simulink model "auv2D_model"  (R2023b)
settings: Solver=FixedStepAuto  StartTime=0.0  StopTime=5  FixedStep=1e-6  RelTol=1e-3
values from neighbouring files (symbols this model uses):
  a1 = Xu/(m-Xud)    (= -0.280372492837)    [auv2D_parameters.m]
  a2 = Yv/(m-Yvd)    (= -0.993417702334)    [auv2D_parameters.m]
  a3 = Nr/(Iz-Nrd)    (= -0.172919127086)    [auv2D_parameters.m]
  b1 = (m-Yvd)/(m-Xud)    (= 2.1006049029)    [auv2D_parameters.m]
  b2 = (Xud-m)/(m-Yvd)    (= -0.4760533495)    [auv2D_parameters.m]
  b3 = (Yvd-Xud)/(Iz-Nrd)    (= -0.887548138639)    [auv2D_parameters.m]
libraries: simulink x1
settings Model: Creator=abinashagasti  LastModifiedBy=abinashagasti

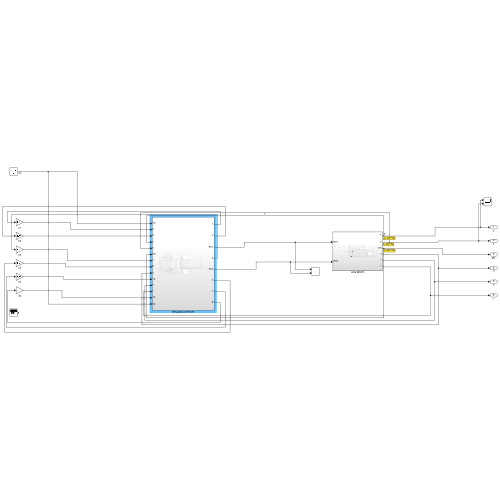
[thumbnail: Simulink's stored preview of the top-level diagram]
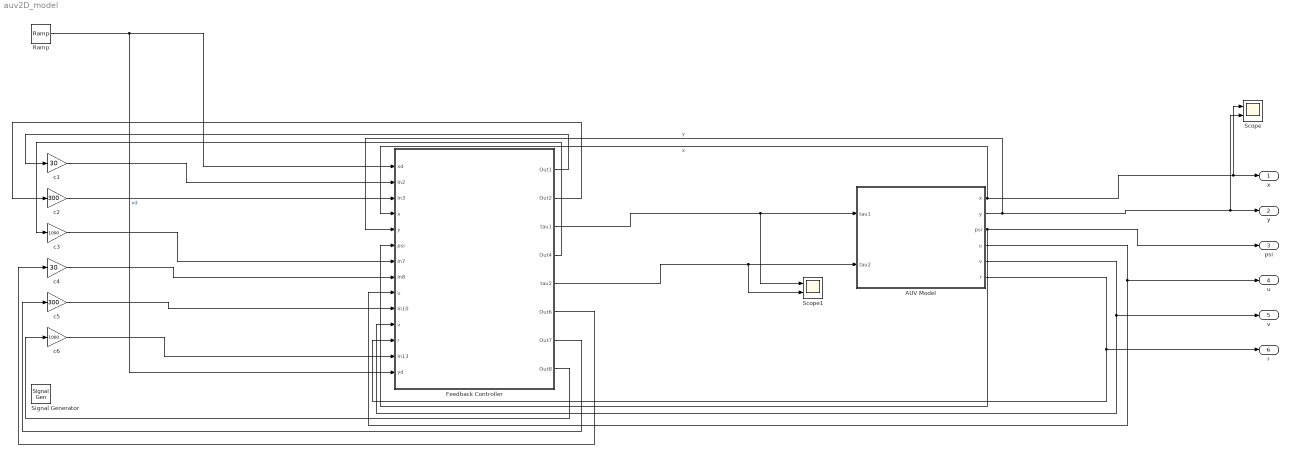
== system auv2D_model ==
  AUV Model : Subsystem
  Feedback Controller : Subsystem
  Ramp : simulink/Sources/Ramp  slope=0.1  start=0  InitialOutput=0
  Scope : Scope  NumInputPorts=2
  Scope1 : Scope  NumInputPorts=2
  Signal Generator : SignalGenerator  Frequency=0.1  Units=rad/sec
  c1 : Gain  Gain=30
  c2 : Gain  Gain=300
  c3 : Gain  Gain=1000
  c4 : Gain  Gain=30
  c5 : Gain  Gain=300
  c6 : Gain  Gain=1000
  x : Outport
  y : Outport  Port=2
  psi : Outport  Port=3
  u : Outport  Port=4
  v : Outport  Port=5
  r : Outport  Port=6
  wires:
  AUV Model/1(x) -> Feedback Controller/4(x), Scope/1, x/1  "x"
  AUV Model/2(y) -> Feedback Controller/5(y), Scope/2, y/1  "y"
  AUV Model/3(psi) -> Feedback Controller/6(psi), psi/1
  AUV Model/4(u) -> Feedback Controller/9(u), u/1
  AUV Model/5(v) -> v/1, Feedback Controller/11(v)
  AUV Model/6(r) -> r/1, Feedback Controller/12(r)
  Ramp/1 -> Feedback Controller/14(yd), Feedback Controller/1(xd)  "xd"
  c1/1 -> Feedback Controller/2(In2)
  c2/1 -> Feedback Controller/3(In3)
  c3/1 -> Feedback Controller/7(In7)
  c4/1 -> Feedback Controller/8(In8)
  c5/1 -> Feedback Controller/10(In10)
  c6/1 -> Feedback Controller/13(In13)
  Feedback Controller/1(Out1) -> c1/1
  Feedback Controller/2(Out2) -> c2/1
  Feedback Controller/3(tau1) -> Scope1/1, AUV Model/1(tau1)
  Feedback Controller/4(Out4) -> c3/1
  Feedback Controller/5(tau2) -> Scope1/2, AUV Model/2(tau2)
  Feedback Controller/6(Out6) -> c4/1
  Feedback Controller/7(Out7) -> c5/1
  Feedback Controller/8(Out8) -> c6/1

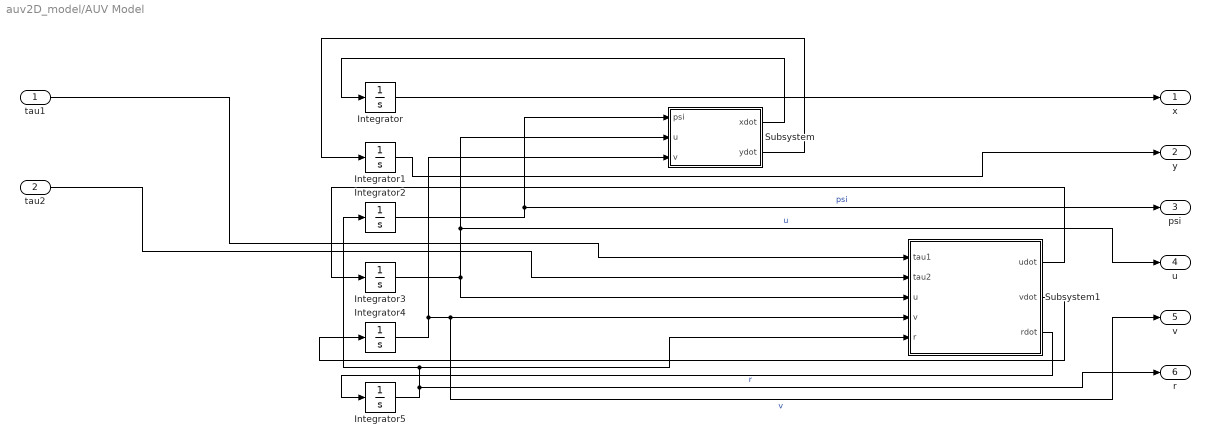
== system auv2D_model/AUV Model ==
  tau1 : Inport
  tau2 : Inport  Port=2
  Integrator{,1,4..5} (4 alike) : Integrator
  Integrator2 : Integrator  InitialCondition=pi/4
  Integrator3 : Integrator  InitialCondition=1
  Subsystem : Subsystem
  Subsystem1 : Subsystem
  x : Outport
  y : Outport  Port=2
  psi : Outport  Port=3
  u : Outport  Port=4
  v : Outport  Port=5
  r : Outport  Port=6
  wires:
  Subsystem1/2(vdot) -> Integrator4/1
  tau2/1 -> Subsystem1/2(tau2)
  Subsystem/2(ydot) -> Integrator1/1
  tau1/1 -> Subsystem1/1(tau1)
  Subsystem1/3(rdot) -> Integrator5/1
  Subsystem1/1(udot) -> Integrator3/1
  Integrator2/1 -> psi/1, Subsystem/1(psi)  "psi"
  Integrator4/1 -> Subsystem/3(v), v/1, Subsystem1/4(v)  "v"
  Integrator1/1 -> y/1
  Subsystem/1(xdot) -> Integrator/1
  Integrator5/1 -> r/1, Subsystem1/5(r), Integrator2/1  "r"
  Integrator/1 -> x/1
  Integrator3/1 -> u/1, Subsystem/2(u), Subsystem1/3(u)  "u"

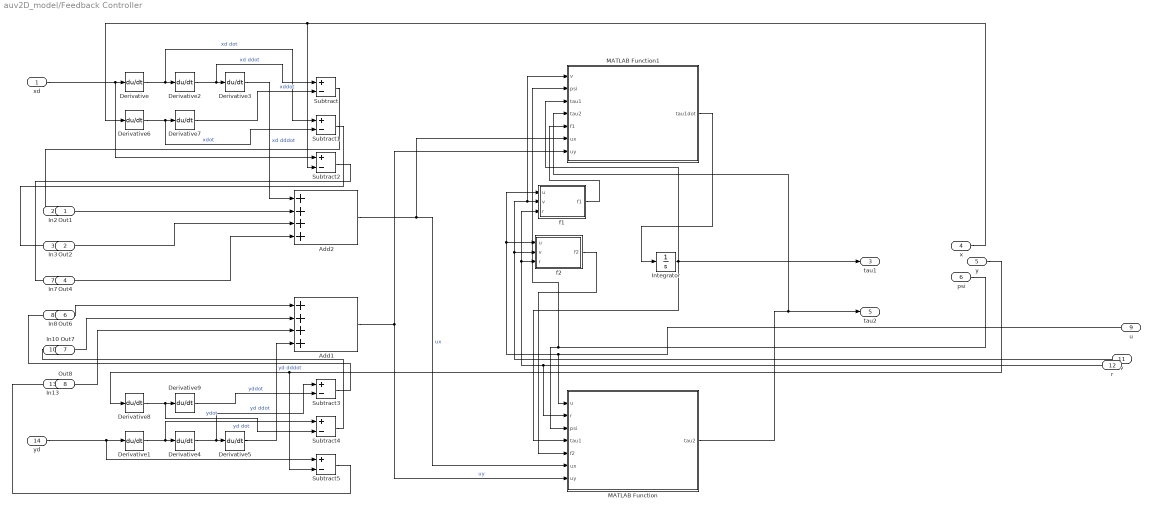
== system auv2D_model/Feedback Controller ==
  xd : Inport
  In2 : Inport  Port=2
  In3 : Inport  Port=3
  x : Inport  Port=4
  y : Inport  Port=5
  psi : Inport  Port=6
  In7 : Inport  Port=7
  In8 : Inport  Port=8
  u : Inport  Port=9
  In10 : Inport  Port=10
  v : Inport  Port=11
  r : Inport  Port=12
  In13 : Inport  Port=13
  yd : Inport  Port=14
  Add1 : Sum  Inputs=++++
  Add2 : Sum  Inputs=++++
  Derivative{,1..9} (10 alike) : Derivative
  Integrator : Integrator
  MATLAB Function : MATLAB Function  TreatAsAtomicUnit=on
  MATLAB Function1 : MATLAB Function  TreatAsAtomicUnit=on
  Subtract{,1..5} (6 alike) : Sum  Inputs=+-
  f1 : MATLAB Function  TreatAsAtomicUnit=on
  f2 : MATLAB Function  TreatAsAtomicUnit=on
  Out1 : Outport
  Out2 : Outport  Port=2
  tau1 : Outport  Port=3
  Out4 : Outport  Port=4
  tau2 : Outport  Port=5
  Out6 : Outport  Port=6
  Out7 : Outport  Port=7
  Out8 : Outport  Port=8
  wires:
  In2/1 -> Add2/2
  Subtract1/1 -> Out2/1
  Subtract4/1 -> Out7/1
  Derivative5/1 -> Add1/4  "yd dddot"
  Derivative7/1 -> Subtract/2  "xddot"
  x/1 -> Subtract2/2, Derivative6/1
  In7/1 -> Add2/4
  Add2/1 -> MATLAB Function1/6(ux), MATLAB Function/6(ux)  "ux"
  Subtract/1 -> Out1/1
  f2/1(f2) -> MATLAB Function/5(f2)
  v/1 -> f2/2(v), MATLAB Function1/1(v), f1/2(v)
  MATLAB Function1/1(tau1dot) -> Integrator/1
  Derivative6/1 -> Subtract1/2, Derivative7/1  "xdot"
  Derivative/1 -> Subtract1/1, Derivative2/1  "xd dot"
  Subtract2/1 -> Out4/1
  In8/1 -> Add1/1
  MATLAB Function/1(tau2) -> tau2/1, MATLAB Function1/4(tau2)
  f1/1(f1) -> MATLAB Function1/5(f1)
  Derivative8/1 -> Subtract4/2, Derivative9/1  "ydot"
  xd/1 -> Subtract2/1, Derivative/1
  Derivative4/1 -> Subtract3/1, Derivative5/1  "yd ddot"
  Subtract3/1 -> Out6/1
  In13/1 -> Add1/3
  In3/1 -> Add2/3
  Derivative1/1 -> Subtract4/1, Derivative4/1  "yd dot"
  Subtract5/1 -> Out8/1
  Integrator/1 -> tau1/1, MATLAB Function1/3(tau1), MATLAB Function/4(tau1)
  r/1 -> MATLAB Function/2(r), f2/3(r), f1/3(r)
  Add1/1 -> MATLAB Function1/7(uy), MATLAB Function/7(uy)  "uy"
  u/1 -> MATLAB Function/1(u), f2/1(u), f1/1(u)
  yd/1 -> Subtract5/1, Derivative1/1
  Derivative3/1 -> Add2/1  "xd dddot"
  In10/1 -> Add1/2
  y/1 -> Subtract5/2, Derivative8/1
  Derivative2/1 -> Subtract/1, Derivative3/1  "xd ddot"
  psi/1 -> MATLAB Function1/2(psi), MATLAB Function/3(psi)
  Derivative9/1 -> Subtract3/2  "yddot"

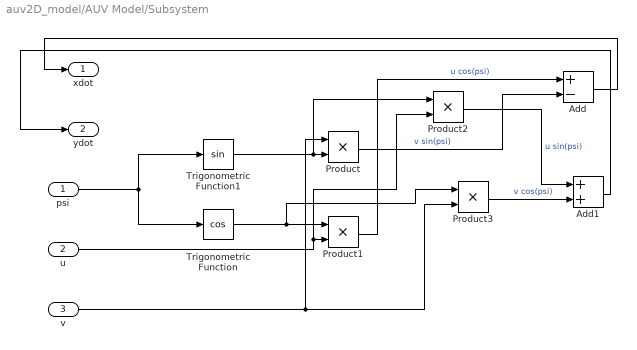
== system auv2D_model/AUV Model/Subsystem ==
  psi : Inport
  u : Inport  Port=2
  v : Inport  Port=3
  Add : Sum  Inputs=+-
  Add1 : Sum
  Product{,1..3} (4 alike) : Product
  Trigonometric Function : Trigonometry  Operator=cos
  Trigonometric Function1 : Trigonometry
  xdot : Outport
  ydot : Outport  Port=2
  wires:
  Add1/1 -> ydot/1
  Product2/1 -> Add1/1  "u sin(psi)"
  Trigonometric Function1/1 -> Product2/1, Product/2
  Product1/1 -> Add/1  "u cos(psi)"
  Product3/1 -> Add1/2  "v cos(psi)"
  v/1 -> Product/1, Product3/2
  Product/1 -> Add/2  "v sin(psi)"
  u/1 -> Product2/2, Product1/2
  Trigonometric Function/1 -> Product3/1, Product1/1
  Add/1 -> xdot/1
  psi/1 -> Trigonometric Function/1, Trigonometric Function1/1

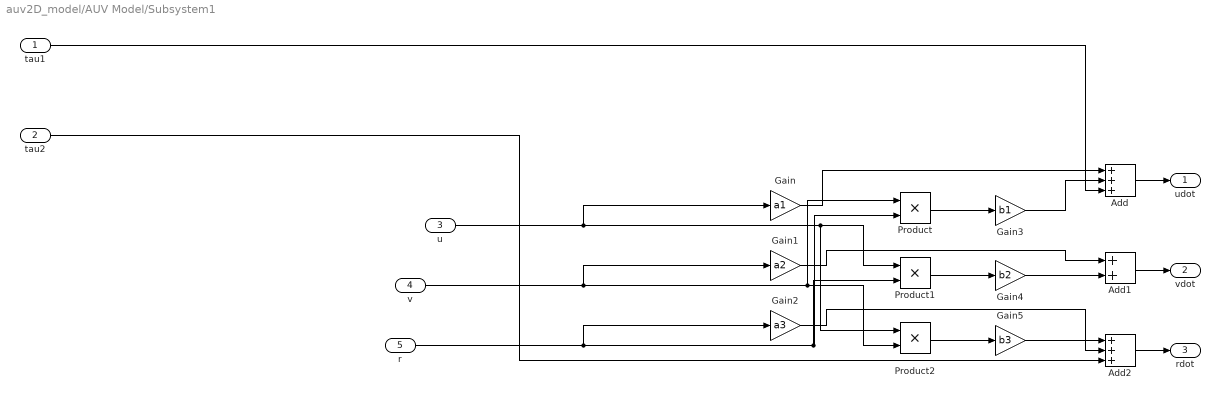
== system auv2D_model/AUV Model/Subsystem1 ==
  tau1 : Inport
  tau2 : Inport  Port=2
  u : Inport  Port=3
  v : Inport  Port=4
  r : Inport  Port=5
  Add : Sum  Inputs=+++
  Add1 : Sum
  Add2 : Sum  Inputs=+++
  Gain : Gain  Gain=a1
  Gain1 : Gain  Gain=a2
  Gain2 : Gain  Gain=a3
  Gain3 : Gain  Gain=b1
  Gain4 : Gain  Gain=b2
  Gain5 : Gain  Gain=b3
  Product : Product
  Product1 : Product
  Product2 : Product
  udot : Outport
  vdot : Outport  Port=2
  rdot : Outport  Port=3
  wires:
  tau2/1 -> Add2/3
  Add1/1 -> vdot/1
  tau1/1 -> Add/3
  u/1 -> Product1/1, Product2/1, Gain/1
  Gain1/1 -> Add1/1
  Product2/1 -> Gain5/1
  v/1 -> Product/1, Product2/2, Gain1/1
  Gain5/1 -> Add2/1
  Add2/1 -> rdot/1
  Gain4/1 -> Add1/2
  Gain3/1 -> Add/2
  Gain/1 -> Add/1
  Gain2/1 -> Add2/2
  r/1 -> Product1/2, Product/2, Gain2/1
  Add/1 -> udot/1
  Product/1 -> Gain3/1
  Product1/1 -> Gain4/1

== matlab function auv2D_model/Feedback Controller/f2 ==
  data: u input; f2 output; v input; r input
function f2 = fcn(u,v,r)

coder.extrinsic('evalin')
a1 = 0;
a1 = evalin('base','a1');
a2 = 0;
a2 = evalin('base','a2');
a3 = 0;
a3 = evalin('base','a3');
b1 = 0;
b1 = evalin('base','b1');
b2 = 0;
b2 = evalin('base','b2');
b3 = 0;
b3 = evalin('base','b3');

f2 = a2^2*v+((a1+a2+a3)*b2+2*a1+a3)*u*r+(b1*b2+2*b1-1)*v*r^2+(b2*b3+b3)*u^2*v;

== matlab function auv2D_model/Feedback Controller/f1 ==
  data: u input; f1 output; v input; r input
function f1 = fcn(u,v,r)
    
coder.extrinsic('evalin')
a1 = 0;
a1 = evalin('base','a1');
a2 = 0;
a2 = evalin('base','a2');
a3 = 0;
a3 = evalin('base','a3');
b1 = 0;
b1 = evalin('base','b1');
b2 = 0;
b2 = evalin('base','b2');
b3 = 0;
b3 = evalin('base','b3');

f1 = a1^2*u+((a1+a2+a3)*b1-2*a2-a3)*v*r+(b1*b2-2*b2-1)*u*r^2+(b1*b3-b3)*u*v^2;

== matlab function auv2D_model/Feedback Controller/MATLAB Function ==
  data: u input; tau2 output; r input; psi input; tau1 input; f2 input; ux input; uy input
function tau2 = fcn(u,r,psi,tau1,f2,ux,uy)

coder.extrinsic('evalin')
a1 = 0;
a1 = evalin('base','a1');
a2 = 0;
a2 = evalin('base','a2');
a3 = 0;
a3 = evalin('base','a3');
b1 = 0;
b1 = evalin('base','b1');
b2 = 0;
b2 = evalin('base','b2');
b3 = 0;
b3 = evalin('base','b3');

tau2 = (1/((b2+1)*u))*(-(b2+2)*r*tau1-f2-ux*sin(psi)+uy*cos(psi));

== matlab function auv2D_model/Feedback Controller/MATLAB Function1 ==
  data: v input; tau1dot output; psi input; tau1 input; tau2 input; f1 input; ux input; uy input
function tau1dot = fcn(v,psi,tau1,tau2,f1,ux,uy)

coder.extrinsic('evalin')
a1 = 0;
a1 = evalin('base','a1');
a2 = 0;
a2 = evalin('base','a2');
a3 = 0;
a3 = evalin('base','a3');
b1 = 0;
b1 = evalin('base','b1');
b2 = 0;
b2 = evalin('base','b2');
b3 = 0;
b3 = evalin('base','b3');

tau1dot = -(a1*tau1+(b1-1)*v*tau2)-f1+ux*cos(psi)+uy*sin(psi);
